simulink model "ideal_model"  (R2021b)
settings: Solver=VariableStepAuto  StartTime=0.0  StopTime=5  MaxStep=1e-5  RelTol=1e-3
libraries: spsMeanLib x9, spsDiodeLib x7, spsACVoltageSourceLib x3, spsVoltageMeasurementLib x3, spsDCVoltageSourceLib x2, spsCurrentMeasurementLib x2, spsSeriesRLCBranchLib x2, spsDCMachineLib x1, spsMosfetLib x1, spsPWMGeneratorDCDCLib x1, eePowerMeasurement x1, spspowerguiLib x1
settings Model: Creator=pc  LastModifiedBy=pc

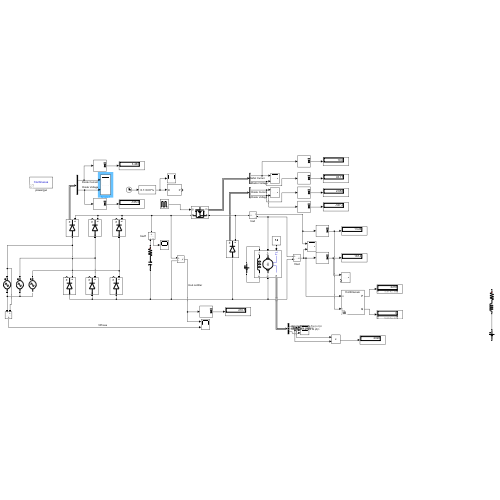
[thumbnail: Simulink's stored preview of the top-level diagram]
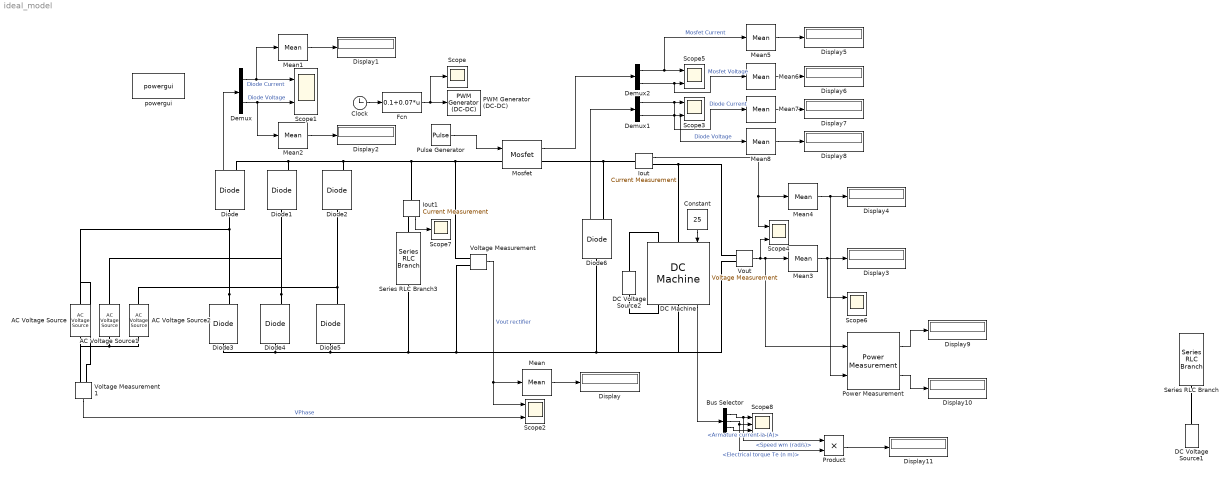
== system ideal_model ==
  AC Voltage Source : spsACVoltageSourceLib/AC Voltage Source  Amplitude=90*sqrt(2)  Phase=0  Frequency=50  SampleTime=0  Measurements=None  BusType=swing  Pref=10e3  Qref=0  Qmin=-inf  Qmax=+inf
  AC Voltage Source1 : spsACVoltageSourceLib/AC Voltage Source  Amplitude=90*sqrt(2)  Phase=-120  Frequency=50  SampleTime=0  Measurements=None  BusType=swing  Pref=10e3  Qref=0  Qmin=-inf  Qmax=+inf
  AC Voltage Source2 : spsACVoltageSourceLib/AC Voltage Source  Amplitude=90*sqrt(2)  Phase=120  Frequency=50  SampleTime=0  Measurements=None  BusType=swing  Pref=10e3  Qref=0  Qmin=-inf  Qmax=+inf
  Bus Selector : BusSelector  OutputSignals=Speed wm (rad/s),Electrical torque Te (n m),Armature current ia (A)
  Clock : Clock
  Constant : Constant  Value=25
  DC Machine : spsDCMachineLib/DC Machine  PresetModel=No  MechanicalLoad=Torque TL  FieldType=Wound  ShowDetailedParameters=on  MeasurementBus=off  RLa="[ 1.07  0.0245]"  RLf="[ 210  23]"  Laf=1.8  MachineConstant=Torque constant (N.m/A)  Ke=1.8  Kt=1.8  J=1  Bm=0  Tf=0  w0=1  Ifinit=1.04761904761905  TsPowergui=0  TsBlock=-1
  DC Voltage Source1 : spsDCVoltageSourceLib/DC Voltage Source  Amplitude=0.1  Measurements=None
  DC Voltage Source2 : spsDCVoltageSourceLib/DC Voltage Source  Amplitude=220  Measurements=None
  Demux : Demux  Outputs=2
  Demux1 : Demux  Outputs=2
  Demux2 : Demux  Outputs=2
  Diode{,1..6} (7 alike) : spsDiodeLib/Diode  Ron=0  Lon=0  Vf=0  IC=0  UseSnubber=0  Rs=inf  Cs=0  Measurements=on
  Display{,1..11} (12 alike) : Display
  Fcn : Fcn  Expr=0.1+0.07*u
  Iout : spsCurrentMeasurementLib/Current Measurement  PhasorSimulation=off  OutputType=Complex  PSBequivalent=0
  Iout1 : spsCurrentMeasurementLib/Current Measurement  PhasorSimulation=off  OutputType=Complex  PSBequivalent=0
  Mean{,1..8} (9 alike) : spsMeanLib/Mean  Freq=50  Vinit=0  Ts=0
  Mosfet : spsMosfetLib/Mosfet  Ron=0.1  Lon=0  Rd=0.01  Vfd=0  IC=0  Rs=1e5  Cs=inf  Measurements=on
  PWM Generator (DC-DC) : spsPWMGeneratorDCDCLib/PWM Generator (DC-DC)  Fsw=1000  Ts=0
  Power Measurement : eePowerMeasurement/Power Measurement  LabelModeActiveChoice=Continuous  F=60  K=[0 1 2 3]  Ts=0
      settings: SourceProductBaseCode=PS
  Product : Product
  Pulse Generator : DiscretePulseGenerator  PulseType=Time based  Period=1/10000  PulseWidth=80
  Scope : Scope
  Scope{1..6} (6 alike) : Scope  NumInputPorts=2
  Scope7 : Scope
  Scope8 : Scope  NumInputPorts=3
  Series RLC Branch : spsSeriesRLCBranchLib/Series RLC Branch  LConnTagsString=__new0  RConnTagsString=__new0  BranchType=RL  Resistance=1.07  Inductance=24e-3  SetiL0=off  InitialCurrent=0  Capacitance=1e-6  Setx0=off  InitialVoltage=0  Measurements=None
  Series RLC Branch3 : spsSeriesRLCBranchLib/Series RLC Branch  LConnTagsString=__new0  RConnTagsString=__new0  BranchType=RC  Resistance=0.0001  Inductance=1e-3  SetiL0=off  InitialCurrent=0  Capacitance=100e-6  Setx0=off  InitialVoltage=0  Measurements=None
  Voltage Measurement : spsVoltageMeasurementLib/Voltage Measurement  PhasorSimulation=off  OutputType=Complex  PSBequivalent=0
  Voltage Measurement1 : spsVoltageMeasurementLib/Voltage Measurement  PhasorSimulation=off  OutputType=Complex  PSBequivalent=0
  Vout : spsVoltageMeasurementLib/Voltage Measurement  PhasorSimulation=off  OutputType=Complex  PSBequivalent=0
  powergui : spspowerguiLib/powergui  Priority=1  SimulationMode=Continuous  SampleTime=50e-6  frequency=60  Iterations=50  frequencyindice=0  Pbase=100e6  ErrMax=1e-4  UnitsV=kV  UnitsW=MW  buscounter=0  FunctionMessages=off  echomessages=off  EnableUseOfTLC=off  CurrentSourceSwitches=off  DisableSnubberDevices=off  DisableRonSwitches=off  DisableVfSwitches=off  DisplayEquations=off  AutomaticDiscreteSolvers=off  SolverType=Tustin/Backward Euler (TBE)  Interpol=off  ExternalGateDelay=off  methode=off  Ts=100  x0status=blocks  SPID=on  SwTol=0  HookPort=off  NonlinearTolerance=1e-4  nMaxIteration=100  ContinueOnMaxIteration=off  RestoreLinks=warning  ResistiveCurrentMeasurement=off  Frange=[0:2:500]  Ylog=off  Xlog=on  ShowGrid=off  save=off  variable=ZData  structure=0  ZoomFFT=off  StartTime=0.0  cycles=1  DisplayStyle=1  fundamental=60  FreqAxis=off  MaxFrequency=1000  frequencyindicesteady=1  RmsSteady=1  display=off
  wires:
  Mosfet/1 -> Demux2/1
  Iout1/1 -> Scope7/1
  Clock/1 -> Fcn/1
  Diode6/1 -> Demux1/1
  Power Measurement/2 -> Display10/1
  Mean3/1 -> Scope6/1, Display3/1
  Mean/1 -> Display/1
  Fcn/1 -> PWM Generator (DC-DC)/1, Scope/1
  Power Measurement/1 -> Display9/1
  Constant/1 -> DC Machine/1
  Mean6/1 -> Display6/1
  Demux1/1 -> Mean7/1, Scope3/1  "Diode Current"
  Demux/1 -> Mean1/1, Scope1/1  "Diode Current"
  Vout/1 -> Scope4/2, Power Measurement/1, Mean3/1
  Mean7/1 -> Display7/1
  Iout/1 -> Mean4/1, Scope4/1
  Mean2/1 -> Display2/1
  Demux2/1 -> Mean5/1, Scope5/1  "Mosfet Current"
  Mean4/1 -> Power Measurement/2, Display4/1
  Demux2/2 -> Mean6/1, Scope5/2  "Mosfet Voltage"
  Mean8/1 -> Display8/1
  Mean1/1 -> Display1/1
  Diode/1 -> Demux/1
  Voltage Measurement/1 -> Scope2/1, Mean/1  "Vout rectifier"
  Demux/2 -> Mean2/1, Scope1/2  "Diode Voltage"
  Voltage Measurement1/1 -> Scope2/2  "VPhase"
  Demux1/2 -> Mean8/1, Scope3/2  "Diode Voltage"
  Mean5/1 -> Display5/1
  Bus Selector/3 -> Scope8/3  "<Armature current ia (A)>"
  Bus Selector/1 -> Product/1, Scope8/1  "<Speed wm (rad/s)>"
  Bus Selector/2 -> Product/2, Scope8/2  "<Electrical torque Te (n m)>"
  Product/1 -> Display11/1
  Pulse Generator/1 -> Mosfet/1
  DC Machine/1 -> Bus Selector/1
  connections:
  AC Voltage Source1/LConn1 -- Voltage Measurement1/LConn2 -- AC Voltage Source/LConn1 -- AC Voltage Source2/LConn1
  Diode4/RConn1 -- Diode1/LConn1 -- AC Voltage Source1/RConn1
  Mosfet/LConn1 -- Diode/RConn1 -- Diode1/RConn1 -- Diode2/RConn1 -- Iout1/LConn1 -- Voltage Measurement/LConn1
  Diode6/RConn1 -- Mosfet/RConn1 -- Iout/LConn1
  AC Voltage Source2/RConn1 -- Diode2/LConn1 -- Diode5/RConn1
  Diode4/LConn1 -- Diode3/LConn1 -- Diode5/LConn1 -- Series RLC Branch3/RConn1 -- DC Machine/RConn1 -- Vout/LConn2 -- Diode6/LConn1 -- Voltage Measurement/LConn2
  Iout/RConn1 -- DC Machine/LConn1 -- Vout/LConn1
  Diode3/RConn1 -- Voltage Measurement1/LConn1 -- AC Voltage Source/RConn1 -- Diode/LConn1
  Series RLC Branch3/LConn1 -- Iout1/RConn1
  DC Voltage Source2/LConn1 -- DC Machine/RConn2
  DC Voltage Source2/RConn1 -- DC Machine/LConn2
  Series RLC Branch/RConn1 -- DC Voltage Source1/RConn1
